simulink subsystem "CrazyflieSensors"  (R2024b)
settings: Solver=VariableStepAuto  StartTime=0.0  StopTime=10.0  RelTol=1e-3
undefined symbols (not defined in the file): a, dspblkCoreblockFVToolHelper, gcbh
settings Model: Creator=luker  LastModifiedBy=luker

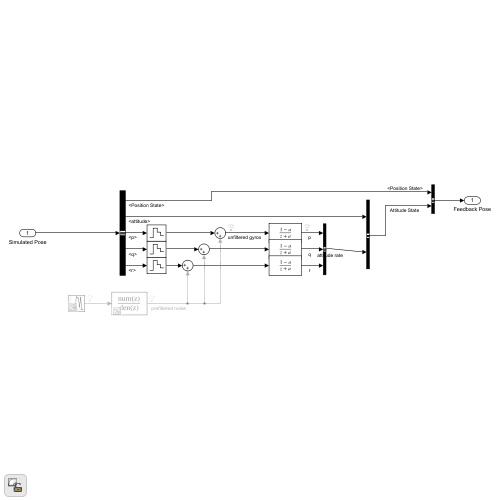
[thumbnail: Simulink's stored preview of the top-level diagram]
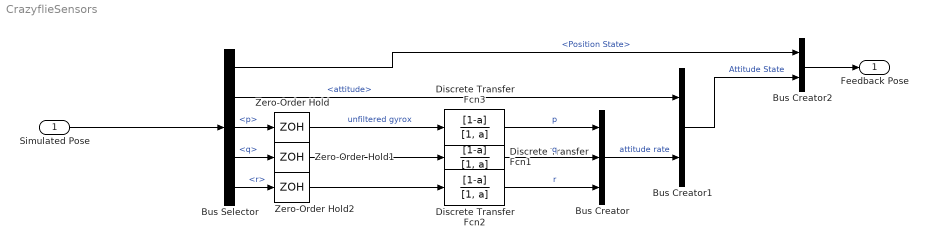
== system CrazyflieSensors ==
  Simulated Pose : Inport
  Bus Creator : BusCreator  Inputs=3
  Bus Creator1 : BusCreator  Inputs=2
  Bus Creator2 : BusCreator  Inputs=2
  Bus Selector : BusSelector  OutputSignals=Position State,Attitude State.attitude,Attitude State.attitude rate.p,Attitude State.attitude rate.q,Attitude State.attitude rate.r
  Discrete Transfer Fcn1 : DiscreteTransferFcn  LoadFcn=dspblkCoreblockFVToolHelper(gcbh,'load');  Numerator=[1-a]  Denominator=[1, a]
      settings: CopyFcn=dspblkCoreblockFVToolHelper(gcbh,'copy');  DeleteFcn=dspblkCoreblockFVToolHelper(gcbh,'close');  ModelCloseFcn=dspblkCoreblockFVToolHelper(gcbh,'close');  PreSaveFcn=dspblkCoreblockFVToolHelper(gcbh,'presave');  PostSaveFcn=dspblkCoreblockFVToolHelper(gcbh,'postsave');  CloseFcn=dspblkCoreblockFVToolHelper(gcbh,'close');
  Discrete Transfer Fcn2 : DiscreteTransferFcn  LoadFcn=dspblkCoreblockFVToolHelper(gcbh,'load');  Numerator=[1-a]  Denominator=[1, a]
      settings: CopyFcn=dspblkCoreblockFVToolHelper(gcbh,'copy');  DeleteFcn=dspblkCoreblockFVToolHelper(gcbh,'close');  ModelCloseFcn=dspblkCoreblockFVToolHelper(gcbh,'close');  PreSaveFcn=dspblkCoreblockFVToolHelper(gcbh,'presave');  PostSaveFcn=dspblkCoreblockFVToolHelper(gcbh,'postsave');  CloseFcn=dspblkCoreblockFVToolHelper(gcbh,'close');
  Discrete Transfer Fcn3 : DiscreteTransferFcn  LoadFcn=dspblkCoreblockFVToolHelper(gcbh,'load');  Numerator=[1-a]  Denominator=[1, a]
      settings: CopyFcn=dspblkCoreblockFVToolHelper(gcbh,'copy');  DeleteFcn=dspblkCoreblockFVToolHelper(gcbh,'close');  ModelCloseFcn=dspblkCoreblockFVToolHelper(gcbh,'close');  PreSaveFcn=dspblkCoreblockFVToolHelper(gcbh,'presave');  PostSaveFcn=dspblkCoreblockFVToolHelper(gcbh,'postsave');  CloseFcn=dspblkCoreblockFVToolHelper(gcbh,'close');
  Zero-Order Hold : ZeroOrderHold  SampleTime=0.001
  Zero-Order Hold1 : ZeroOrderHold  SampleTime=0.001
  Zero-Order Hold2 : ZeroOrderHold  SampleTime=0.001
  Feedback Pose : Outport
  wires:
  Simulated Pose/1 -> Bus Selector/1
  Bus Selector/5 -> Zero-Order Hold2/1  "<r>"
  Bus Selector/4 -> Zero-Order Hold1/1  "<q>"
  Bus Selector/3 -> Zero-Order Hold/1  "<p>"
  Zero-Order Hold/1 -> Discrete Transfer Fcn3/1  "unfiltered gyrox"
  Zero-Order Hold1/1 -> Discrete Transfer Fcn1/1
  Zero-Order Hold2/1 -> Discrete Transfer Fcn2/1
  Bus Creator/1 -> Bus Creator1/2  "attitude rate"
  Bus Selector/2 -> Bus Creator1/1  "<attitude>"
  Bus Creator1/1 -> Bus Creator2/2  "Attitude State"
  Bus Selector/1 -> Bus Creator2/1  "<Position State>"
  Bus Creator2/1 -> Feedback Pose/1
  Discrete Transfer Fcn3/1 -> Bus Creator/1  "p"
  Discrete Transfer Fcn1/1 -> Bus Creator/2  "q"
  Discrete Transfer Fcn2/1 -> Bus Creator/3  "r"
